simulink model "plant"  (R2015a)
settings: Solver=FixedStepDiscrete  StartTime=0.0  StopTime=10.0  RelTol=1e-3
values from neighbouring files (symbols this model uses):
  A = [3.29698189006 1 0 0 -4.20791026518 0 1 0 2.48348543348 0 0 1 ... (16 elements, 4x4)]    [end_of_class.mat]    (also in log_observer_test.mat; parameters.mat)
  B = [1 0 0 0]    [end_of_class.mat]    (also in log_observer_test.mat; parameters.mat)
  C = [-0.0495309545297 0.081302844811 0.0308276179144 0]    [end_of_class.mat]    (also in log_observer_test.mat; parameters.mat)
settings Model: Creator=alunos  LastModifiedBy=hdplsa
settings DataIOCC: LimitDataPoints=off

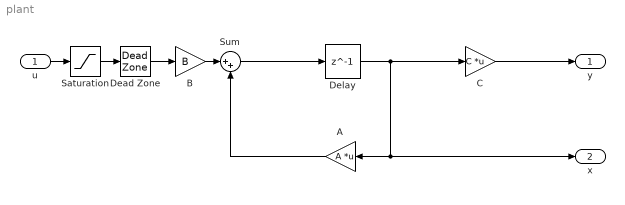
== system plant ==
  u : Inport
  A : Gain  Gain=A  Multiplication=Matrix(K*u)
  B : Gain  Gain=B
  C : Gain  Gain=C  Multiplication=Matrix(K*u)
  Dead Zone : DeadZone  LowerValue=-0.17  UpperValue=0.45  SaturateOnIntegerOverflow=on
  Delay : Delay  DelayLength=1  InitialCondition=[0;0;0;0]
  Saturation : Saturate  UpperLimit=5  LowerLimit=-5
  Sum : Sum  Inputs=|++
  y : Outport
  x : Outport  Port=2
  wires:
  u/1 -> Saturation/1
  C/1 -> y/1
  Delay/1 -> x/1, A/1, C/1
  B/1 -> Sum/1
  Sum/1 -> Delay/1
  A/1 -> Sum/2
  Saturation/1 -> Dead Zone/1
  Dead Zone/1 -> B/1
